simulink model "CubeStacking"  (R2024a)
settings: Solver=VariableStepDiscrete  StartTime=0.0  StopTime=inf  RelTol=1e-3
libraries: simulink x6, ros2lib x2, rllib x1
settings Model: Creator=cgpda  LastModifiedBy=mikel
settings OptimizationCC: EnhancedBackFolding=on  PassReuseOutputArgsAs=Individual arguments  ZeroExternalMemoryAtStartup=off  ZeroInternalMemoryAtStartup=off  MaxStackSize=64  OptimizeBlockOrder=speed  DifferentSizesBufferReuse=on  OptimizationCustomize=off  EfficientTunableParamExpr=on
settings DebuggingCC: ParameterTunabilityLossMsg=error
settings HardwareCC: ProdBitPerLong=64  ProdHWDeviceType=Intel->x86-64 (Linux 64)
settings SFSimCC: MATLABDynamicMemAlloc=off
settings RTWCC: Description=Embedded Coder  SystemTargetFile=ert.tlc  HardwareBoard=Robot Operating System 2 (ROS 2)  TLCOptions="-aInlineSetEventsForThisBaseRateFcn=TLC_FALSE -aSuppressMultiTaskScheduler=TLC_FALSE  -aRateBasedStepFcn=0"  TemplateMakefile=ert_default_tmf  Toolchain=Colcon Tools  TargetLang=C++  GPUComputeCapability=3.5
settings CodeAppCC: ForceParamTrailComments=on  IgnoreCustomStorageClasses=off  OperatorAnnotations=on  SimulinkDataObjDesc=on  SFDataObjDesc=on  InsertBlockDesc=on
settings ERTTargetCC: CodeInterfacePackaging=C++ class  RootIOFormat=Structure reference

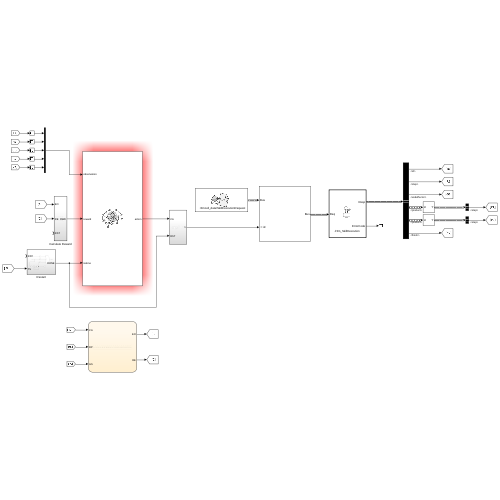
[thumbnail: Simulink's stored preview of the top-level diagram]
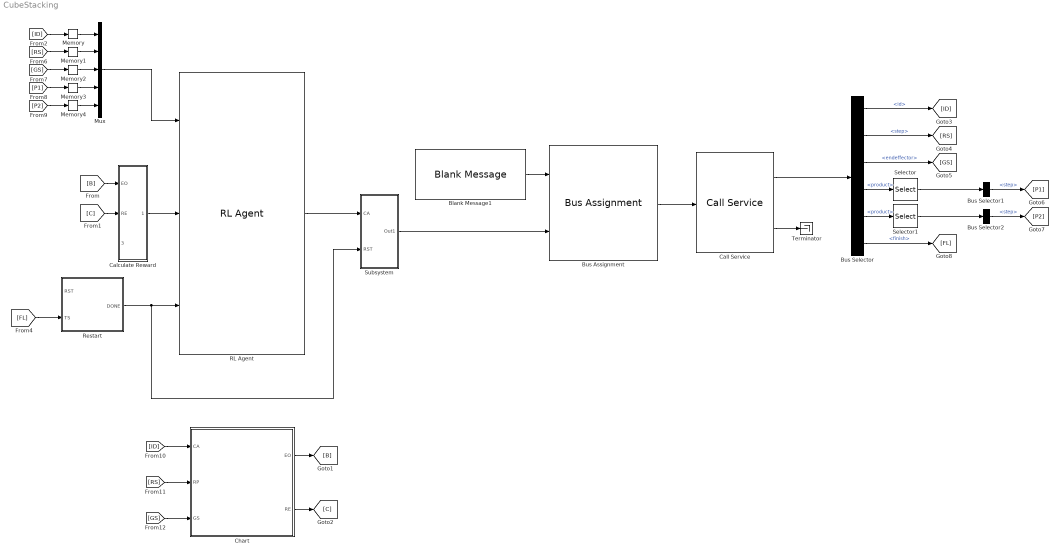
== system CubeStacking ==
  Blank Message1 : ros2lib/Blank Message  messageClass=Service Request  entityType=r3mcell_data/SkillExecution  messageType=r3mcell_data/SkillExecutionRequest  SampleTime=-1
  Bus Assignment : BusAssignment  AssignedSignals=id
  Bus Selector : BusSelector  OutputSignals=result.id,result.robstate.step,result.robstate.endeffector,result.product,result.product,result.finish
  Bus Selector1 : BusSelector  OutputSignals=step
  Bus Selector2 : BusSelector  OutputSignals=step
  Calculate Reward : Subsystem
  Call Service : ros2lib/Call Service  topicSource=Select from ROS network  service=/r3m_SkillExecution  serviceType=r3mcell_data/SkillExecution  connectionTimeout=5  ShowErrorCodeOutput=on  legacyBusStruct=off  QOSHistory=Keep last  QOSDepth=1  QOSReliability=Reliable  QOSDurability=Volatile  QOSDeadline=Inf  QOSLifespan=Inf  QOSLiveliness=Automatic  QOSLeaseDuration=Inf  QOSAvoidROSNamespaceConventions=off
  Chart : Stateflow chart  TreatAsAtomicUnit=on
  Memory : Memory  InitialCondition=1
  Memory1 : Memory  InitialCondition=1
  Memory2 : Memory  InitialCondition=1
  Memory3 : Memory
  Memory4 : Memory
  Mux : Mux  Inputs=5
  RL Agent : rllib/RL Agent  Agent=agent1  ExternalActionAsInput=off  ProvideLastAction=off  ProvideCumRwd=off  TreatAsDirectFeedthrough=on  UseStrictObservationDataTypes=off
  Restart : Subsystem
  Selector : Selector  InputPortWidth=16  IndexOptions=Index vector (dialog)  Indices=[1]  OutputSizes=1
  Selector1 : Selector  InputPortWidth=16  IndexOptions=Index vector (dialog)  Indices=[2]  OutputSizes=1
  Subsystem : Subsystem
  Terminator : Terminator
  wires:
  Restart/1(DONE) -> Subsystem/2(RST), RL Agent/3
  Calculate Reward/1(RWD) -> RL Agent/2
  [FL] -> Restart/2(TS)
  Mux/1 -> RL Agent/1
  [B] -> Calculate Reward/1(EO)
  [C] -> Calculate Reward/2(RE)
  Chart/1(EO) -> [B]
  Chart/2(RE) -> [C]
  Blank Message1/1 -> Bus Assignment/1
  Call Service/1 -> Bus Selector/1
  Bus Assignment/1 -> Call Service/1
  Call Service/2 -> Terminator/1
  [P2] -> Memory4/1
  [P1] -> Memory3/1
  [GS] -> Memory2/1
  [RS] -> Memory1/1
  [ID] -> Memory/1
  [ID] -> Chart/1(CA)
  [RS] -> Chart/2(RP)
  [GS] -> Chart/3(GS)
  Subsystem/1(Out1) -> Bus Assignment/2
  RL Agent/1 -> Subsystem/1(CA)
  Memory/1 -> Mux/1
  Memory1/1 -> Mux/2
  Memory2/1 -> Mux/3
  Memory3/1 -> Mux/4
  Memory4/1 -> Mux/5
  Bus Selector/1 -> [ID]  "<id>"
  Bus Selector/2 -> [RS]  "<step>"
  Bus Selector/3 -> [GS]  "<endeffector>"
  Bus Selector/6 -> [FL]  "<finish>"
  Bus Selector/4 -> Selector/1  "<product>"
  Bus Selector/5 -> Selector1/1  "<product>"
  Selector/1 -> Bus Selector1/1
  Bus Selector1/1 -> [P1]  "<step>"
  Selector1/1 -> Bus Selector2/1
  Bus Selector2/1 -> [P2]  "<step>"

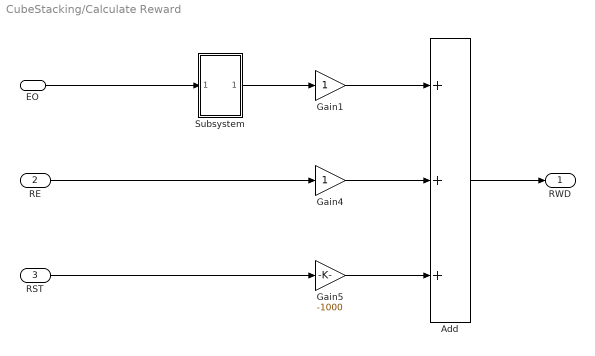
== system CubeStacking/Calculate Reward ==
  EO : Inport
  RE : Inport  Port=2
  RST : Inport  Port=3
  Add : Sum  Inputs=+++
  Gain1 : Gain
  Gain4 : Gain
  Gain5 : Gain  Gain=-1000
  Subsystem : Subsystem
  RWD : Outport
  wires:
  Add/1 -> RWD/1
  RST/1 -> Gain5/1
  Gain5/1 -> Add/3
  Gain1/1 -> Add/1
  EO/1 -> Subsystem/1(In1)
  Subsystem/1(Out1) -> Gain1/1
  Gain4/1 -> Add/2
  RE/1 -> Gain4/1

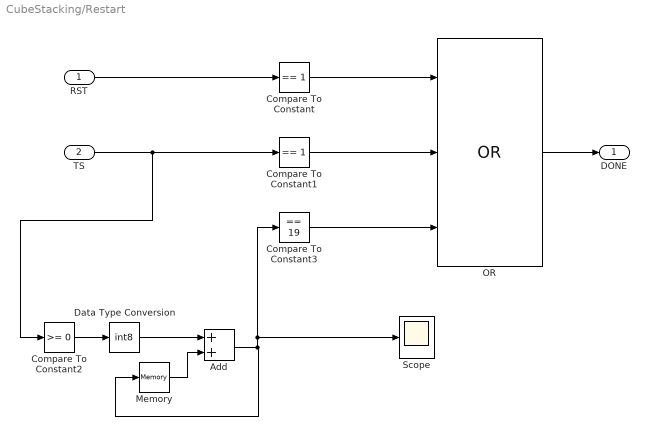
== system CubeStacking/Restart ==
  RST : Inport
  TS : Inport  Port=2
  Add : Sum
  Compare To Constant : simulink/Logic and Bit Operations/Compare To Constant  relop===  const=1  OutDataTypeStr=boolean
  Compare To Constant1 : simulink/Logic and Bit Operations/Compare To Constant  relop===  const=1  OutDataTypeStr=boolean
  Compare To Constant2 : simulink/Logic and Bit Operations/Compare To Constant  relop=>=  const=0  OutDataTypeStr=boolean
  Compare To Constant3 : simulink/Logic and Bit Operations/Compare To Constant  relop===  const=19  OutDataTypeStr=boolean
  Data Type Conversion : DataTypeConversion  OutDataTypeStr=int8  SaturateOnIntegerOverflow=off  RndMeth=Floor
  Memory : Memory
  OR : Logic  Operator=OR  Inputs=3  IconShape=distinctive  AllPortsSameDT=off  OutDataTypeStr=boolean
  Scope : Scope
  DONE : Outport
  wires:
  OR/1 -> DONE/1
  Compare To Constant/1 -> OR/1
  Compare To Constant1/1 -> OR/2
  RST/1 -> Compare To Constant/1
  TS/1 -> Compare To Constant2/1, Compare To Constant1/1
  Compare To Constant2/1 -> Data Type Conversion/1
  Memory/1 -> Add/2
  Data Type Conversion/1 -> Add/1
  Add/1 -> Compare To Constant3/1, Scope/1, Memory/1
  Compare To Constant3/1 -> OR/3

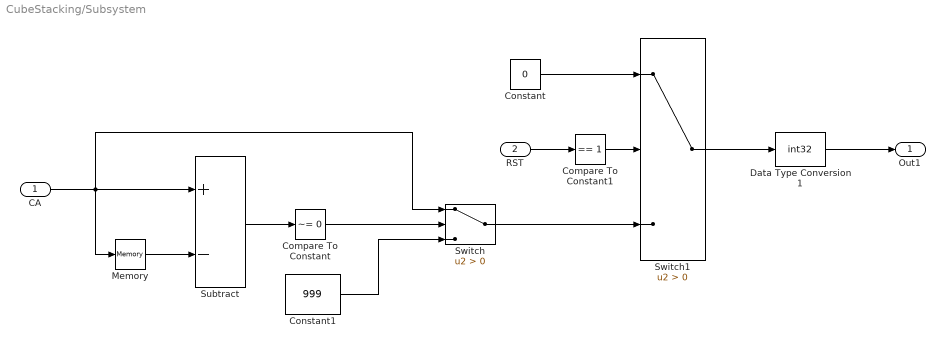
== system CubeStacking/Subsystem ==
  CA : Inport
  RST : Inport  Port=2
  Compare To Constant : simulink/Logic and Bit Operations/Compare To Constant  relop=~=  const=0  OutDataTypeStr=boolean
  Compare To Constant1 : simulink/Logic and Bit Operations/Compare To Constant  relop===  const=1  OutDataTypeStr=boolean
  Constant : Constant  Value=0  SampleTime=-1
  Constant1 : Constant  Value=999  SampleTime=-1
  Data Type Conversion1 : DataTypeConversion  OutMin=[0]  OutMax=[7]  OutDataTypeStr=int32  SaturateOnIntegerOverflow=off  RndMeth=Floor
  Memory : Memory  InheritSampleTime=on
  Subtract : Sum  Inputs=+-
  Switch : Switch  Criteria=u2 > Threshold  SaturateOnIntegerOverflow=off  InputSameDT=off
  Switch1 : Switch  Criteria=u2 > Threshold  SaturateOnIntegerOverflow=off  InputSameDT=off
  Out1 : Outport
  wires:
  Subtract/1 -> Compare To Constant/1
  Memory/1 -> Subtract/2
  Data Type Conversion1/1 -> Out1/1
  Constant1/1 -> Switch/3
  Compare To Constant/1 -> Switch/2
  CA/1 -> Switch/1, Subtract/1, Memory/1
  Switch1/1 -> Data Type Conversion1/1
  RST/1 -> Compare To Constant1/1
  Compare To Constant1/1 -> Switch1/2
  Switch/1 -> Switch1/3
  Constant/1 -> Switch1/1

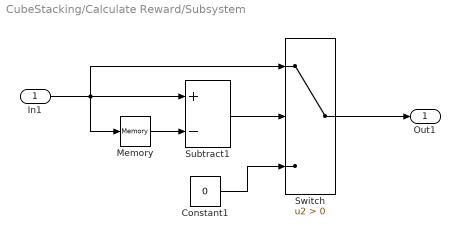
== system CubeStacking/Calculate Reward/Subsystem ==
  In1 : Inport
  Constant1 : Constant  Value=0
  Memory : Memory
  Subtract1 : Sum  Inputs=+-
  Switch : Switch  Criteria=u2 > Threshold  SaturateOnIntegerOverflow=off  InputSameDT=off
  Out1 : Outport
  wires:
  Memory/1 -> Subtract1/2
  Constant1/1 -> Switch/3
  Subtract1/1 -> Switch/2
  In1/1 -> Memory/1, Switch/1, Subtract1/1
  Switch/1 -> Out1/1

== stateflow chart CubeStacking/Chart ==
  state ProductRequirements2 [parallel]
    settings: executionOrder=1
    state RecipeError1
      entry, during:
      RE=-500;
    state RecipeError2
      entry, during:
      RE=-500;
    state RecipeError3
      entry, during:
      RE=-500;
    state RecipeError4
      entry, during:
      RE=-500;
    state RecipeError5
      entry, during:
      RE=-500;
    state RecipeError6
      entry, during:
      RE=-500;
    state RecipeError7
      entry, during:
      RE=-500;
    state RecipeError8
      entry, during:
      RE=-500;
    state RecipeError9
      entry, during:
      RE=-500;
    state RecipeError15
      entry, during:
      RE=-500;
    state RecipeError10
      entry, during:
      RE=-500;
    state RecipeError11
      entry, during:
      RE=-500;
    state RecipeError14
      entry, during:
      RE=-500;
    state RecipeError13
      entry, during:
      RE=-500;
    state RecipeError12
      entry, during:
      RE=-500;
    state RecipeError16
      entry, during:
      RE=-500;
    state RecipeError17
      entry, during:
      RE=-500;
    state RecipeError18
      entry, during:
      RE=-500;
    state ProductInitialState
      entry, during:
      RE=0; EO=0;
    state SkillReq1Completed
      entry, during:
      RE=0; EO=100;
    state SkillReq2Completed
      entry, during:
      RE=0; EO=200;
    state SkillReq3Completed
      entry, during:
      RE=0; EO=300;
    state SkillReq4Completed
      entry, during:
      RE=0; EO=400;
    state SkillReq5Completed
      entry, during:
      RE=0; EO=500;
    state SkillReq6Completed
      entry, during:
      RE=0; EO=600
    state SkillReq7Completed
      entry, during:
      RE=0; EO=700;
    state SkillReq8Completed
      entry, during:
      RE=0; EO=800;
    state SkillReq9Completed
      entry, during:
      RE=0; EO=900;
    state SkillReq1Completed1
      entry, during:
      RE=0; EO=1000;
    state SkillReq2Completed1
      entry, during:
      RE=0; EO=1100;
    state SkillReq3Completed1
      entry, during:
      RE=0; EO=1200;
    state SkillReq4Completed1
      entry, during:
      RE=0; EO=1300;
    state SkillReq5Completed1
      entry, during:
      RE=0; EO=1400;
    state SkillReq6Completed1
      entry, during:
      RE=0; EO=1500
    state SkillReq7Completed1
      entry, during:
      RE=0; EO=1600;
    state SkillReq8Completed1
      entry, during:
      RE=0; EO=1700;
    state SkillReq9Completed1
      entry, during:
      RE=0; EO=1800;
    ProductInitialState -> RecipeError1 [order 2] : [CA~=2]
    SkillReq1Completed -> RecipeError2 [order 2] : [CA~=3]
    SkillReq2Completed -> RecipeError3 [order 2] : [CA~=6]
    SkillReq3Completed -> RecipeError4 [order 2] : [CA~=2]
    SkillReq4Completed -> RecipeError5 [order 2] : [CA~=4]
    SkillReq6Completed -> RecipeError7 [order 2] : [CA~=7]
    SkillReq7Completed -> RecipeError8 [order 2] : [CA~=4]
    SkillReq8Completed -> RecipeError9 [order 2] : [CA~=1]
    SkillReq9Completed -> RecipeError15 [order 2] : [CA~=12]
    SkillReq1Completed1 -> RecipeError10 [order 2] : [CA~=13]
    SkillReq2Completed1 -> RecipeError11 [order 2] : [CA~=6]
    SkillReq3Completed1 -> RecipeError14 [order 2] : [CA~=12]
    SkillReq4Completed1 -> RecipeError13 [order 2] : [CA~=14]
    SkillReq6Completed1 -> RecipeError16 [order 2] : [CA~=7]
    SkillReq7Completed1 -> RecipeError17 [order 2] : [CA~=14]
    SkillReq8Completed1 -> RecipeError18 [order 2] : [CA~=1]
    SkillReq5Completed -> RecipeError6 [order 2] : [CA~=5]
    SkillReq5Completed1 -> RecipeError12 [order 2] : [CA~=15]
    RecipeError1 -> SkillReq1Completed : [RP==2 && GS==1]
    RecipeError2 -> SkillReq2Completed : [RP==3 && GS==1]
    RecipeError3 -> SkillReq3Completed : [RP==3 && GS==0]
    RecipeError4 -> SkillReq4Completed : [RP==2 && GS==0]
    RecipeError5 -> SkillReq5Completed : [RP==4 && GS==0]
    RecipeError6 -> SkillReq6Completed : [RP==5 && GS==0]
    RecipeError7 -> SkillReq7Completed : [RP==5 && GS==1]
    RecipeError8 -> SkillReq8Completed : [RP==4 && GS==1]
    RecipeError9 -> SkillReq9Completed : [RP==1 && GS==1]
    RecipeError15 -> SkillReq1Completed1 : [RP==12 && GS==1]
    RecipeError10 -> SkillReq2Completed1 : [RP==13 && GS==1]
    RecipeError11 -> SkillReq3Completed1 : [RP==13 && GS==0]
    RecipeError14 -> SkillReq4Completed1 : [RP==12 && GS==0]
    RecipeError13 -> SkillReq5Completed1 : [RP==14 && GS==0]
    RecipeError12 -> SkillReq6Completed1 : [RP==15 && GS==0]
    RecipeError16 -> SkillReq7Completed1 : [RP==15 && GS==1]
    RecipeError17 -> SkillReq8Completed1 : [RP==14 && GS==1]
    RecipeError18 -> SkillReq9Completed1 : [RP==1 && GS==1]
    (default) -> ProductInitialState
    SkillReq5Completed -> SkillReq6Completed [order 1] : [CA==5]
    SkillReq5Completed1 -> SkillReq6Completed1 [order 1] : [CA==15]
    SkillReq7Completed -> SkillReq8Completed [order 1] : [CA==4]
    SkillReq8Completed -> SkillReq9Completed [order 1] : [CA==1]
    SkillReq9Completed -> SkillReq1Completed1 [order 1] : [CA==12]
    SkillReq7Completed1 -> SkillReq8Completed1 [order 1] : [CA==14]
    SkillReq8Completed1 -> SkillReq9Completed1 [order 1] : [CA==1]
    SkillReq1Completed -> SkillReq2Completed [order 1] : [CA==3]
    SkillReq1Completed1 -> SkillReq2Completed1 [order 1] : [CA==13]
    ProductInitialState -> SkillReq1Completed [order 1] : [CA==2]
    SkillReq2Completed -> SkillReq3Completed [order 1] : [CA==6]
    SkillReq2Completed1 -> SkillReq3Completed1 [order 1] : [CA==6]
    SkillReq4Completed -> SkillReq5Completed [order 1] : [CA==4]
    SkillReq4Completed1 -> SkillReq5Completed1 [order 1] : [CA==14]
    SkillReq3Completed -> SkillReq4Completed [order 1] : [CA==2]
    SkillReq3Completed1 -> SkillReq4Completed1 [order 1] : [CA==12]
    SkillReq6Completed -> SkillReq7Completed [order 1] : [CA==7]
    SkillReq6Completed1 -> SkillReq7Completed1 [order 1] : [CA==7]
  data: EO output; RE output; CA input; RP input; GS input
